simulink model "ball_and_plate_za_nn_2"  (R2018b)
settings: Solver=ode45  StartTime=0.0  StopTime=t_sim  RelTol=1e-3  EnableMultiTasking=on
values from neighbouring files (symbols this model uses):
  A_x = 0.05    [parametri.mat]    (also in proba_nn_simulink.m = 0.1; simulate_NOE_NARX_performance.mat = 0.1; simuliraj_kruznicu.m = radijus; test_nn_.m = 0.1)
  a_x = 0.388    [parametri.mat]    (also in simulate_NOE_NARX_performance.mat)
  A_y = 0.05    [parametri.mat]    (also in proba_nn_simulink.m = 0.1; simulate_NOE_NARX_performance.mat = 0.1; simuliraj_kruznicu.m = radijus; test_nn_.m = 0.1)
  a_y = 0.473    [parametri.mat]    (also in simulate_NOE_NARX_performance.mat)
  Ak_x = 0.1    [parametri.mat]    (also in simulate_NOE_NARX_performance.mat; simuliraj_kvadrat.m = stranica)
  Ak_y = 0.1    [parametri.mat]    (also in simulate_NOE_NARX_performance.mat; simuliraj_kvadrat.m = stranica)
  d = 2    [parametri.mat]    (also in simulate_NOE_NARX_performance.mat)
  Fc = 9.9675e-08    [parametri.mat]    (also in simulate_NOE_NARX_performance.mat)
  freq_x = 0.628318530718    [parametri.mat]    (also in simulate_NOE_NARX_performance.mat)
  freq_y = 0.628318530718    [parametri.mat]    (also in simulate_NOE_NARX_performance.mat)
  Fs = 1.9935e-07    [parametri.mat]    (also in simulate_NOE_NARX_performance.mat)
  g = 9.81    [parametri.mat]    (also in simulate_NOE_NARX_performance.mat)
  Jl = 7.48815837481e-05    [parametri.mat]    (also in simulate_NOE_NARX_performance.mat)
  konstanta = 0.1    [parametri.mat]    (also in simulate_NOE_NARX_performance.mat; simuliraj_kvadrat.m = 0.03)
  l = 0.1    [parametri.mat]    (also in simulate_NOE_NARX_performance.mat)
  ml = 0.0786597330257    [parametri.mat]    (also in simulate_NOE_NARX_performance.mat)
  odabir = 3    [proba_nn_simulink.m]    (also in simulate_NOE_NARX_performance.mat; simuliraj_kruznicu.m; simuliraj_kvadrat.m = 2; simuliraj_referenca.m = 1)
  period_x = 16    [parametri.mat]    (also in simulate_NOE_NARX_performance.mat)
  period_y = 16    [parametri.mat]    (also in simulate_NOE_NARX_performance.mat)
  phase_x = 1.57079632679    [parametri.mat]    (also in simulate_NOE_NARX_performance.mat)
  phase_y = 0    [parametri.mat]    (also in simulate_NOE_NARX_performance.mat)
  phasedelay_x = 0    [parametri.mat]    (also in simulate_NOE_NARX_performance.mat)
  phasedelay_y = 4    [parametri.mat]    (also in simulate_NOE_NARX_performance.mat)
  pw_x = 50    [parametri.mat]    (also in simulate_NOE_NARX_performance.mat)
  pw_y = 50    [parametri.mat]    (also in simulate_NOE_NARX_performance.mat)
  R = 0.0397    [parametri.mat]    (also in simulate_NOE_NARX_performance.mat)
  r = 0.02    [parametri.mat]    (also in simulate_NOE_NARX_performance.mat)
  t_step = 5    [parametri.mat]    (also in simulate_NOE_NARX_performance.mat)
  Td = 0.1    [parametri.mat]    (also in simulate_NOE_NARX_performance.mat)
  vs = 0.05    [parametri.mat]    (also in simulate_NOE_NARX_performance.mat)
  x0 = 0.15    [parametri.mat]    (also in proba_nn_simulink.m = a_x/2.0; simulate_NOE_NARX_performance.mat = 0.194; simuliraj_kruznicu.m = a_x/2.0; test_nn_.m = a_x/2.0)
  x0_loptica = 0.1    [proba_nn_simulink.m]    (also in simulate_NOE_NARX_performance.mat; simuliraj_kruznicu.m = x0_poc; simuliraj_kvadrat.m = x0_poc; simuliraj_referenca.m = x0_poc)
  x_step = 0.05    [parametri.mat]    (also in simulate_NOE_NARX_performance.mat; simuliraj_referenca.m = x_ref_value)
  y0 = 0.15    [parametri.mat]    (also in proba_nn_simulink.m = a_y/2.0; simulate_NOE_NARX_performance.mat = 0.2365; simuliraj_kruznicu.m = a_y/2.0; test_nn_.m = a_y/2.0)
  y0_loptica = 0.1    [proba_nn_simulink.m]    (also in simulate_NOE_NARX_performance.mat; simuliraj_kruznicu.m = y0_poc; simuliraj_kvadrat.m = y0_poc; simuliraj_referenca.m = y0_poc)
  y_step = 0.05    [parametri.mat]    (also in simulate_NOE_NARX_performance.mat; simuliraj_referenca.m = y_ref_value)
libraries: neural x118, simulink x6, fuzblock x2
(part 4 of 5)

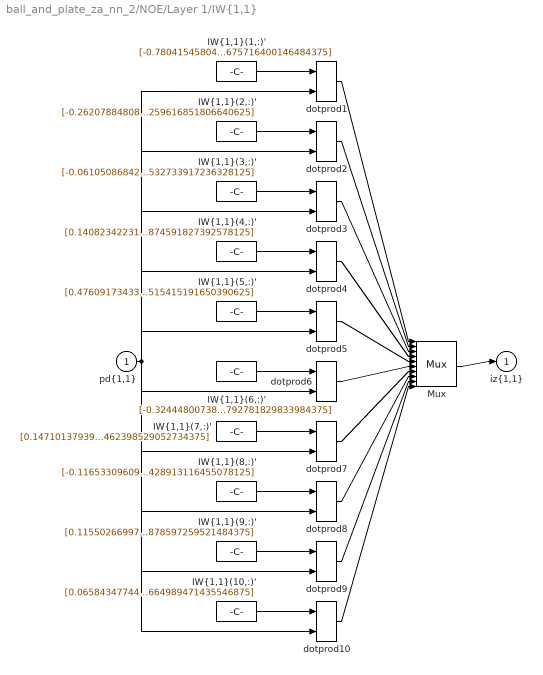
== system ball_and_plate_za_nn_2/NOE/Layer 1/IW{1,1} ==
  "pd{1,1}" : Inport  PortDimensions=5  SampleTime=0.001
      mask Display: e = 0.06;c1 = [120 230 180]/255;c2 = ([120 230 180]+0)/(256+128);c3 = ([120 230 180]+128)/(256+128);patch([0 1 1 0],[0 0 1 1],c1);patch([0 1 1 1-e 1-e 0+e],[0 0 1 1-e 0+e 0+e],c2);patch([0 0 1 1-e 0+e 0+e],[0 1 1 1-e 1-e 0+e],c3);plot([0 1 1 0 0],[0 0 1 1 0]);
  "IW{1,1}(1,:)'" : Constant  Value=[-0.78041545804284273568640628582215867936611175537109375;-0.1889168057158937263917408699853694997727870941162109375;0.624203755586431707769179411116056144237518310546875;0.38254385586967643018141416177968494594097137451171875;0.11132858481816297613331556703997193835675716400146484375]
      mask Display: e = 0.06;c1 = [120 150 230]/255;c2 = ([120 150 230]+0)/383;c3 = ([120 150 230]+128)/383;patch([0 1 1 0],[0 0 1 1],c1);patch([0 1 1 1-e 1-e 0+e],[0 0 1 1-e 0+e 0+e],c2);patch([0 0 1 1-e 0+e 0+e],[0 1 1 1-e 1-e 0+e],c3);plot([0 1 1 0 0],[0 0 1 1 0]);disp('Weights');
  "IW{1,1}(10,:)'" : Constant  Value=[0.06584347744638797961247433931930572725832462310791015625;-0.14742080631494014486548849163227714598178863525390625;-0.449429553740740950207310788755421526730060577392578125;-0.10537733622991619919506689484478556551039218902587890625;0.57322556196782226134445181742194108664989471435546875]
      mask Display: e = 0.06;c1 = [120 150 230]/255;c2 = ([120 150 230]+0)/383;c3 = ([120 150 230]+128)/383;patch([0 1 1 0],[0 0 1 1],c1);patch([0 1 1 1-e 1-e 0+e],[0 0 1 1-e 0+e 0+e],c2);patch([0 0 1 1-e 0+e 0+e],[0 1 1 1-e 1-e 0+e],c3);plot([0 1 1 0 0],[0 0 1 1 0]);disp('Weights');
  "IW{1,1}(2,:)'" : Constant  Value=[-0.26207884808871162451993086506263352930545806884765625;0.06367181522086796940929076527027064003050327301025390625;0.06797795577746899853277540159979253076016902923583984375;0.469471262437006375822790005258866585791110992431640625;0.196872246361272262848984837546595372259616851806640625]
      mask Display: e = 0.06;c1 = [120 150 230]/255;c2 = ([120 150 230]+0)/383;c3 = ([120 150 230]+128)/383;patch([0 1 1 0],[0 0 1 1],c1);patch([0 1 1 1-e 1-e 0+e],[0 0 1 1-e 0+e 0+e],c2);patch([0 0 1 1-e 0+e 0+e],[0 1 1 1-e 1-e 0+e],c3);plot([0 1 1 0 0],[0 0 1 1 0]);disp('Weights');
  "IW{1,1}(3,:)'" : Constant  Value=[-0.06105086842811814629161659695455455221235752105712890625;0.4362035008337665775712821414344944059848785400390625;0.4757244892843950356819959779386408627033233642578125;-0.332950625751637419025286135365604422986507415771484375;-0.1849610518275301984658653964288532733917236328125]
      mask Display: e = 0.06;c1 = [120 150 230]/255;c2 = ([120 150 230]+0)/383;c3 = ([120 150 230]+128)/383;patch([0 1 1 0],[0 0 1 1],c1);patch([0 1 1 1-e 1-e 0+e],[0 0 1 1-e 0+e 0+e],c2);patch([0 0 1 1-e 0+e 0+e],[0 1 1 1-e 1-e 0+e],c3);plot([0 1 1 0 0],[0 0 1 1 0]);disp('Weights');
  "IW{1,1}(4,:)'" : Constant  Value=[0.1408234223110425842317994238328537903726100921630859375;-0.13205465366012736350143086383468471467494964599609375;-0.493931339703755745151880773846642114222049713134765625;-0.2126283255869568511453593373516923747956752777099609375;-0.12407140487677166540425588436846737749874591827392578125]
      mask Display: e = 0.06;c1 = [120 150 230]/255;c2 = ([120 150 230]+0)/383;c3 = ([120 150 230]+128)/383;patch([0 1 1 0],[0 0 1 1],c1);patch([0 1 1 1-e 1-e 0+e],[0 0 1 1-e 0+e 0+e],c2);patch([0 0 1 1-e 0+e 0+e],[0 1 1 1-e 1-e 0+e],c3);plot([0 1 1 0 0],[0 0 1 1 0]);disp('Weights');
  "IW{1,1}(5,:)'" : Constant  Value=[0.476091734332447114041997338063083589076995849609375;-0.63150999375165917104624213607166893780231475830078125;-0.515564815245219687511735173757188022136688232421875;-0.1465624758355017487332361270091496407985687255859375;0.2165017929034026844536953149145119823515415191650390625]
      mask Display: e = 0.06;c1 = [120 150 230]/255;c2 = ([120 150 230]+0)/383;c3 = ([120 150 230]+128)/383;patch([0 1 1 0],[0 0 1 1],c1);patch([0 1 1 1-e 1-e 0+e],[0 0 1 1-e 0+e 0+e],c2);patch([0 0 1 1-e 0+e 0+e],[0 1 1 1-e 1-e 0+e],c3);plot([0 1 1 0 0],[0 0 1 1 0]);disp('Weights');
  "IW{1,1}(6,:)'" : Constant  Value=[-0.324448007382350411820226554482360370457172393798828125;-0.166002451601267642100623334044939838349819183349609375;0.297221055954937696252926571105490438640117645263671875;0.380975071646488083754178433082415722310543060302734375;-0.233386025845927436161986179286031983792781829833984375]
      mask Display: e = 0.06;c1 = [120 150 230]/255;c2 = ([120 150 230]+0)/383;c3 = ([120 150 230]+128)/383;patch([0 1 1 0],[0 0 1 1],c1);patch([0 1 1 1-e 1-e 0+e],[0 0 1 1-e 0+e 0+e],c2);patch([0 0 1 1-e 0+e 0+e],[0 1 1 1-e 1-e 0+e],c3);plot([0 1 1 0 0],[0 0 1 1 0]);disp('Weights');
  "IW{1,1}(7,:)'" : Constant  Value=[0.1471013793978408756846221194791723974049091339111328125;-0.039050046429146945126120726854423992335796356201171875;0.441337535111876066995506562307127751410007476806640625;0.1489052345501019336548864657743251882493495941162109375;0.01257927307039984066161508735604002140462398529052734375]
      mask Display: e = 0.06;c1 = [120 150 230]/255;c2 = ([120 150 230]+0)/383;c3 = ([120 150 230]+128)/383;patch([0 1 1 0],[0 0 1 1],c1);patch([0 1 1 1-e 1-e 0+e],[0 0 1 1-e 0+e 0+e],c2);patch([0 0 1 1-e 0+e 0+e],[0 1 1 1-e 1-e 0+e],c3);plot([0 1 1 0 0],[0 0 1 1 0]);disp('Weights');
  "IW{1,1}(8,:)'" : Constant  Value=[-0.11653309609751634490226734897078131325542926788330078125;0.377889179667925290129204540789942257106304168701171875;0.2200242920649362332596865599043667316436767578125;-0.07683035892270144440185930534426006488502025604248046875;0.462132111220164620846162506495602428913116455078125]
      mask Display: e = 0.06;c1 = [120 150 230]/255;c2 = ([120 150 230]+0)/383;c3 = ([120 150 230]+128)/383;patch([0 1 1 0],[0 0 1 1],c1);patch([0 1 1 1-e 1-e 0+e],[0 0 1 1-e 0+e 0+e],c2);patch([0 0 1 1-e 0+e 0+e],[0 1 1 1-e 1-e 0+e],c3);plot([0 1 1 0 0],[0 0 1 1 0]);disp('Weights');
  "IW{1,1}(9,:)'" : Constant  Value=[0.11550266997215274944466045781155116856098175048828125;0.387383375581388078590094892206252552568912506103515625;-0.62457516979531668699365809516166336834430694580078125;-0.0744787101351869207377376369549892842769622802734375;0.83112863904779332724359619533061049878597259521484375]
      mask Display: e = 0.06;c1 = [120 150 230]/255;c2 = ([120 150 230]+0)/383;c3 = ([120 150 230]+128)/383;patch([0 1 1 0],[0 0 1 1],c1);patch([0 1 1 1-e 1-e 0+e],[0 0 1 1-e 0+e 0+e],c2);patch([0 0 1 1-e 0+e 0+e],[0 1 1 1-e 1-e 0+e],c3);plot([0 1 1 0 0],[0 0 1 1 0]);disp('Weights');
  Mux : Mux  Inputs=10
      mask Display: e = 0.06;c1 = [120 150 230]/255;c2 = ([120 150 230]+0)/383;c3 = ([120 150 230]+128)/383;patch([0 1 1 0],[0 0 1 1],c1);patch([0 1 1 1-e 1-e 0+e],[0 0 1 1-e 0+e 0+e],c2);patch([0 0 1 1-e 0+e 0+e],[0 1 1 1-e 1-e 0+e],c3);plot([0 1 1 0 0],[0 0 1 1 0]);disp('Mux');
  dotprod{1..10} (10 alike) : neural/Weight Functions/dotprod
  "iz{1,1}" : Outport
      mask Display: e = 0.06;c1 = [120 230 180]/255;c2 = ([120 230 180]+0)/(256+128);c3 = ([120 230 180]+128)/(256+128);patch([0 1 1 0],[0 0 1 1],c1);patch([0 1 1 1-e 1-e 0+e],[0 0 1 1-e 0+e 0+e],c2);patch([0 0 1 1-e 0+e 0+e],[0 1 1 1-e 1-e 0+e],c3);plot([0 1 1 0 0],[0 0 1 1 0]);
  wires:
  "IW{1,1}(1,:)'"/1 -> dotprod1/1
  "pd{1,1}"/1 -> dotprod1/2, dotprod2/2, dotprod3/2, dotprod4/2, dotprod5/2, dotprod6/2, dotprod7/2, dotprod8/2, dotprod9/2, dotprod10/2
  dotprod1/1 -> Mux/1
  "IW{1,1}(2,:)'"/1 -> dotprod2/1
  dotprod2/1 -> Mux/2
  "IW{1,1}(3,:)'"/1 -> dotprod3/1
  dotprod3/1 -> Mux/3
  "IW{1,1}(4,:)'"/1 -> dotprod4/1
  dotprod4/1 -> Mux/4
  "IW{1,1}(5,:)'"/1 -> dotprod5/1
  dotprod5/1 -> Mux/5
  "IW{1,1}(6,:)'"/1 -> dotprod6/1
  dotprod6/1 -> Mux/6
  "IW{1,1}(7,:)'"/1 -> dotprod7/1
  dotprod7/1 -> Mux/7
  "IW{1,1}(8,:)'"/1 -> dotprod8/1
  dotprod8/1 -> Mux/8
  "IW{1,1}(9,:)'"/1 -> dotprod9/1
  dotprod9/1 -> Mux/9
  "IW{1,1}(10,:)'"/1 -> dotprod10/1
  dotprod10/1 -> Mux/10
  Mux/1 -> "iz{1,1}"/1

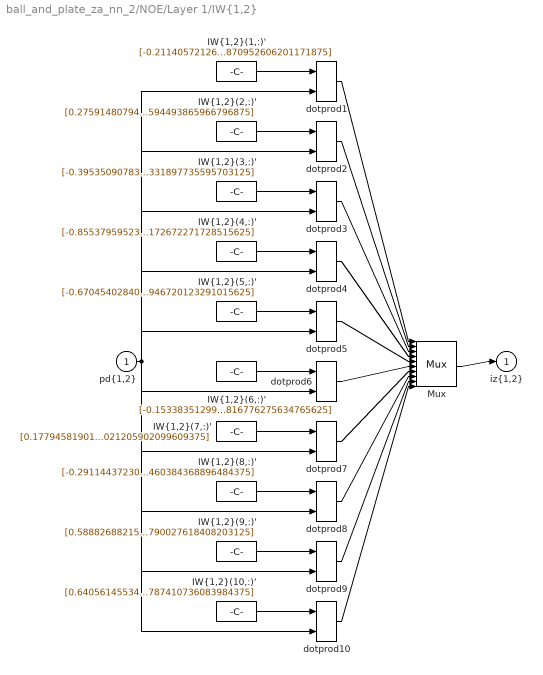
== system ball_and_plate_za_nn_2/NOE/Layer 1/IW{1,2} ==
  "pd{1,2}" : Inport  PortDimensions=5  SampleTime=0.001
      mask Display: e = 0.06;c1 = [120 230 180]/255;c2 = ([120 230 180]+0)/(256+128);c3 = ([120 230 180]+128)/(256+128);patch([0 1 1 0],[0 0 1 1],c1);patch([0 1 1 1-e 1-e 0+e],[0 0 1 1-e 0+e 0+e],c2);patch([0 0 1 1-e 0+e 0+e],[0 1 1 1-e 1-e 0+e],c3);plot([0 1 1 0 0],[0 0 1 1 0]);
  "IW{1,2}(1,:)'" : Constant  Value=[-0.211405721260622792012640047687455080449581146240234375;0.9834201495236669643418281339108943939208984375;0.078318433789418495649670148850418627262115478515625;0.62573603116239862043101993549498729407787322998046875;-0.4606972890689788879825528056244365870952606201171875]
      mask Display: e = 0.06;c1 = [120 150 230]/255;c2 = ([120 150 230]+0)/383;c3 = ([120 150 230]+128)/383;patch([0 1 1 0],[0 0 1 1],c1);patch([0 1 1 1-e 1-e 0+e],[0 0 1 1-e 0+e 0+e],c2);patch([0 0 1 1-e 0+e 0+e],[0 1 1 1-e 1-e 0+e],c3);plot([0 1 1 0 0],[0 0 1 1 0]);disp('Weights');
  "IW{1,2}(10,:)'" : Constant  Value=[0.64056145534157327148250260506756603717803955078125;0.600565723799352024769859781372360885143280029296875;0.2156582058706855153928927393280901014804840087890625;0.6943897986555647161566184877301566302776336669921875;-0.60339661147887768688491405555396340787410736083984375]
      mask Display: e = 0.06;c1 = [120 150 230]/255;c2 = ([120 150 230]+0)/383;c3 = ([120 150 230]+128)/383;patch([0 1 1 0],[0 0 1 1],c1);patch([0 1 1 1-e 1-e 0+e],[0 0 1 1-e 0+e 0+e],c2);patch([0 0 1 1-e 0+e 0+e],[0 1 1 1-e 1-e 0+e],c3);plot([0 1 1 0 0],[0 0 1 1 0]);disp('Weights');
  "IW{1,2}(2,:)'" : Constant  Value=[0.2759148079449758039771722906152717769145965576171875;-0.42325449718057639447721385295153595507144927978515625;-0.1532778579257629003596008487875224091112613677978515625;-0.482010946294399167388888827190385200083255767822265625;-0.664216850422650662011392341810278594493865966796875]
      mask Display: e = 0.06;c1 = [120 150 230]/255;c2 = ([120 150 230]+0)/383;c3 = ([120 150 230]+128)/383;patch([0 1 1 0],[0 0 1 1],c1);patch([0 1 1 1-e 1-e 0+e],[0 0 1 1-e 0+e 0+e],c2);patch([0 0 1 1-e 0+e 0+e],[0 1 1 1-e 1-e 0+e],c3);plot([0 1 1 0 0],[0 0 1 1 0]);disp('Weights');
  "IW{1,2}(3,:)'" : Constant  Value=[-0.39535090783148596482732273216242901980876922607421875;0.0030548046006235456302502218051131421816535294055938720703125;-0.381754713214691510092535509102162905037403106689453125;-0.137371181736283987095958991631050594151020050048828125;-0.54520998452879265716575218903017230331897735595703125]
      mask Display: e = 0.06;c1 = [120 150 230]/255;c2 = ([120 150 230]+0)/383;c3 = ([120 150 230]+128)/383;patch([0 1 1 0],[0 0 1 1],c1);patch([0 1 1 1-e 1-e 0+e],[0 0 1 1-e 0+e 0+e],c2);patch([0 0 1 1-e 0+e 0+e],[0 1 1 1-e 1-e 0+e],c3);plot([0 1 1 0 0],[0 0 1 1 0]);disp('Weights');
  "IW{1,2}(4,:)'" : Constant  Value=[-0.85537959523864859345820832459139637649059295654296875;-0.003498486669252578139255316358458003378473222255706787109375;0.229525682886273785232589261795510537922382354736328125;-0.69954557852212229107635721447877585887908935546875;0.003780760113263581002895907801075736642815172672271728515625]
      mask Display: e = 0.06;c1 = [120 150 230]/255;c2 = ([120 150 230]+0)/383;c3 = ([120 150 230]+128)/383;patch([0 1 1 0],[0 0 1 1],c1);patch([0 1 1 1-e 1-e 0+e],[0 0 1 1-e 0+e 0+e],c2);patch([0 0 1 1-e 0+e 0+e],[0 1 1 1-e 1-e 0+e],c3);plot([0 1 1 0 0],[0 0 1 1 0]);disp('Weights');
  "IW{1,2}(5,:)'" : Constant  Value=[-0.6704540284077300515974684458342380821704864501953125;-0.1356854228754304225734728106544935144484043121337890625;-0.668394792329869869007552551920525729656219482421875;0.44352275149486819483257704632706008851528167724609375;0.1269145397078425274717261572732240892946720123291015625]
      mask Display: e = 0.06;c1 = [120 150 230]/255;c2 = ([120 150 230]+0)/383;c3 = ([120 150 230]+128)/383;patch([0 1 1 0],[0 0 1 1],c1);patch([0 1 1 1-e 1-e 0+e],[0 0 1 1-e 0+e 0+e],c2);patch([0 0 1 1-e 0+e 0+e],[0 1 1 1-e 1-e 0+e],c3);plot([0 1 1 0 0],[0 0 1 1 0]);disp('Weights');
  "IW{1,2}(6,:)'" : Constant  Value=[-0.153383512992241455297204311136738397181034088134765625;-0.1582862661763130562864176908988156355917453765869140625;-0.2420745637484461865174267813927144743502140045166015625;-0.574128226120135476406858288100920617580413818359375;-0.60140197031635145297201461289660073816776275634765625]
      mask Display: e = 0.06;c1 = [120 150 230]/255;c2 = ([120 150 230]+0)/383;c3 = ([120 150 230]+128)/383;patch([0 1 1 0],[0 0 1 1],c1);patch([0 1 1 1-e 1-e 0+e],[0 0 1 1-e 0+e 0+e],c2);patch([0 0 1 1-e 0+e 0+e],[0 1 1 1-e 1-e 0+e],c3);plot([0 1 1 0 0],[0 0 1 1 0]);disp('Weights');
  "IW{1,2}(7,:)'" : Constant  Value=[0.1779458190130129568995442923551308922469615936279296875;0.79003871229958788635627797702909447252750396728515625;0.4392010876973493349595401014084927737712860107421875;0.51372629645238532258844088573823682963848114013671875;0.2078732017274463605982504077474004589021205902099609375]
      mask Display: e = 0.06;c1 = [120 150 230]/255;c2 = ([120 150 230]+0)/383;c3 = ([120 150 230]+128)/383;patch([0 1 1 0],[0 0 1 1],c1);patch([0 1 1 1-e 1-e 0+e],[0 0 1 1-e 0+e 0+e],c2);patch([0 0 1 1-e 0+e 0+e],[0 1 1 1-e 1-e 0+e],c3);plot([0 1 1 0 0],[0 0 1 1 0]);disp('Weights');
  "IW{1,2}(8,:)'" : Constant  Value=[-0.29114437230780498833127012403565458953380584716796875;-0.7687057090658928615312106558121740818023681640625;0.1507041762917487315309728046486270613968372344970703125;-0.3169104871757533192777600561385042965412139892578125;0.475119755527989739984917605397640727460384368896484375]
      mask Display: e = 0.06;c1 = [120 150 230]/255;c2 = ([120 150 230]+0)/383;c3 = ([120 150 230]+128)/383;patch([0 1 1 0],[0 0 1 1],c1);patch([0 1 1 1-e 1-e 0+e],[0 0 1 1-e 0+e 0+e],c2);patch([0 0 1 1-e 0+e 0+e],[0 1 1 1-e 1-e 0+e],c3);plot([0 1 1 0 0],[0 0 1 1 0]);disp('Weights');
  "IW{1,2}(9,:)'" : Constant  Value=[0.58882688215316736357607396712410263717174530029296875;-0.10413231615864219914424637636329862289130687713623046875;0.16252337571316655129294304060749709606170654296875;0.2493172541404560238476051381439901888370513916015625;-1.0104188868762673525480977332335896790027618408203125]
      mask Display: e = 0.06;c1 = [120 150 230]/255;c2 = ([120 150 230]+0)/383;c3 = ([120 150 230]+128)/383;patch([0 1 1 0],[0 0 1 1],c1);patch([0 1 1 1-e 1-e 0+e],[0 0 1 1-e 0+e 0+e],c2);patch([0 0 1 1-e 0+e 0+e],[0 1 1 1-e 1-e 0+e],c3);plot([0 1 1 0 0],[0 0 1 1 0]);disp('Weights');
  Mux : Mux  Inputs=10
      mask Display: e = 0.06;c1 = [120 150 230]/255;c2 = ([120 150 230]+0)/383;c3 = ([120 150 230]+128)/383;patch([0 1 1 0],[0 0 1 1],c1);patch([0 1 1 1-e 1-e 0+e],[0 0 1 1-e 0+e 0+e],c2);patch([0 0 1 1-e 0+e 0+e],[0 1 1 1-e 1-e 0+e],c3);plot([0 1 1 0 0],[0 0 1 1 0]);disp('Mux');
  dotprod{1..10} (10 alike) : neural/Weight Functions/dotprod
  "iz{1,2}" : Outport
      mask Display: e = 0.06;c1 = [120 230 180]/255;c2 = ([120 230 180]+0)/(256+128);c3 = ([120 230 180]+128)/(256+128);patch([0 1 1 0],[0 0 1 1],c1);patch([0 1 1 1-e 1-e 0+e],[0 0 1 1-e 0+e 0+e],c2);patch([0 0 1 1-e 0+e 0+e],[0 1 1 1-e 1-e 0+e],c3);plot([0 1 1 0 0],[0 0 1 1 0]);
  wires:
  "IW{1,2}(1,:)'"/1 -> dotprod1/1
  "pd{1,2}"/1 -> dotprod1/2, dotprod2/2, dotprod3/2, dotprod4/2, dotprod5/2, dotprod6/2, dotprod7/2, dotprod8/2, dotprod9/2, dotprod10/2
  dotprod1/1 -> Mux/1
  "IW{1,2}(2,:)'"/1 -> dotprod2/1
  dotprod2/1 -> Mux/2
  "IW{1,2}(3,:)'"/1 -> dotprod3/1
  dotprod3/1 -> Mux/3
  "IW{1,2}(4,:)'"/1 -> dotprod4/1
  dotprod4/1 -> Mux/4
  "IW{1,2}(5,:)'"/1 -> dotprod5/1
  dotprod5/1 -> Mux/5
  "IW{1,2}(6,:)'"/1 -> dotprod6/1
  dotprod6/1 -> Mux/6
  "IW{1,2}(7,:)'"/1 -> dotprod7/1
  dotprod7/1 -> Mux/7
  "IW{1,2}(8,:)'"/1 -> dotprod8/1
  dotprod8/1 -> Mux/8
  "IW{1,2}(9,:)'"/1 -> dotprod9/1
  dotprod9/1 -> Mux/9
  "IW{1,2}(10,:)'"/1 -> dotprod10/1
  dotprod10/1 -> Mux/10
  Mux/1 -> "iz{1,2}"/1

== system ball_and_plate_za_nn_2/NOE/Layer 2/Delays 1 ==
  "p{2}" : Inport  PortDimensions=10  SampleTime=0.001
      mask Display: e = 0.06;c1 = [120 230 180]/255;c2 = ([120 230 180]+0)/(256+128);c3 = ([120 230 180]+128)/(256+128);patch([0 1 1 0],[0 0 1 1],c1);patch([0 1 1 1-e 1-e 0+e],[0 0 1 1-e 0+e 0+e],c2);patch([0 0 1 1-e 0+e 0+e],[0 1 1 1-e 1-e 0+e],c3);plot([0 1 1 0 0],[0 0 1 1 0]);
  mux : Mux  Inputs=1
      mask Display: e = 0.06;c1 = [120 150 230]/255;c2 = ([120 150 230]+0)/383;c3 = ([120 150 230]+128)/383;patch([0 1 1 0],[0 0 1 1],c1);patch([0 1 1 1-e 1-e 0+e],[0 0 1 1-e 0+e 0+e],c2);patch([0 0 1 1-e 0+e 0+e],[0 1 1 1-e 1-e 0+e],c3);plot([0 1 1 0 0],[0 0 1 1 0]);disp('Mux')
  "pd{2,1}" : Outport
      mask Display: e = 0.06;c1 = [120 230 180]/255;c2 = ([120 230 180]+0)/(256+128);c3 = ([120 230 180]+128)/(256+128);patch([0 1 1 0],[0 0 1 1],c1);patch([0 1 1 1-e 1-e 0+e],[0 0 1 1-e 0+e 0+e],c2);patch([0 0 1 1-e 0+e 0+e],[0 1 1 1-e 1-e 0+e],c3);plot([0 1 1 0 0],[0 0 1 1 0]);
  wires:
  "p{2}"/1 -> mux/1
  mux/1 -> "pd{2,1}"/1

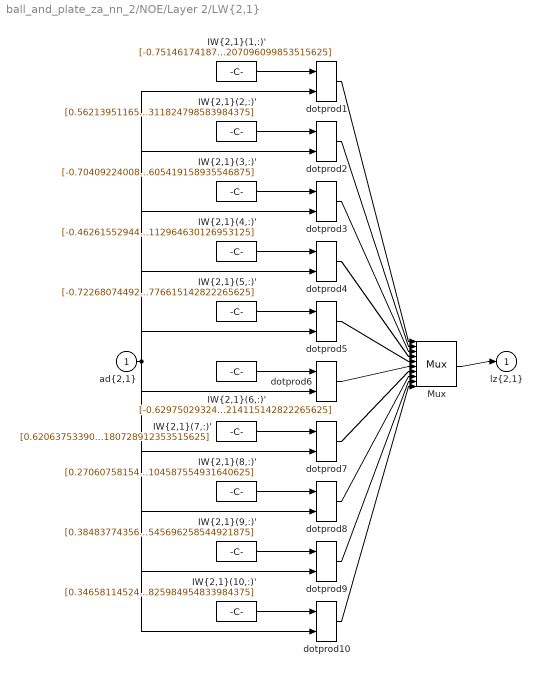
== system ball_and_plate_za_nn_2/NOE/Layer 2/LW{2,1} ==
  "ad{2,1}" : Inport  PortDimensions=10  SampleTime=0.001
      mask Display: e = 0.06;c1 = [120 230 180]/255;c2 = ([120 230 180]+0)/(256+128);c3 = ([120 230 180]+128)/(256+128);patch([0 1 1 0],[0 0 1 1],c1);patch([0 1 1 1-e 1-e 0+e],[0 0 1 1-e 0+e 0+e],c2);patch([0 0 1 1-e 0+e 0+e],[0 1 1 1-e 1-e 0+e],c3);plot([0 1 1 0 0],[0 0 1 1 0]);
  "IW{2,1}(1,:)'" : Constant  Value=[-0.751461741877256894639458550955168902873992919921875;0.01402301635471886638584226858483816613443195819854736328125;0.326442792203841147813392353782546706497669219970703125;0.90660022935466921811809015707694925367832183837890625;-0.407952329174343153450621457523084245622158050537109375;0.609601578751406858458494752994738519191741943359375;-0.255621626399888779435087826641392894089221954345703125;0.10066722871003118411348253857795498333871364593505859375;0.64998266078069499851466161999269388616085052490234375;0.0938512522285636363594818476485670544207096099853515625]
      mask Display: e = 0.06;c1 = [120 150 230]/255;c2 = ([120 150 230]+0)/383;c3 = ([120 150 230]+128)/383;patch([0 1 1 0],[0 0 1 1],c1);patch([0 1 1 1-e 1-e 0+e],[0 0 1 1-e 0+e 0+e],c2);patch([0 0 1 1-e 0+e 0+e],[0 1 1 1-e 1-e 0+e],c3);plot([0 1 1 0 0],[0 0 1 1 0]);disp('weights');
  "IW{2,1}(10,:)'" : Constant  Value=[0.346581145248940847292118405675864778459072113037109375;-0.101987596917314904398921271422295831143856048583984375;-0.199988337664544435501312591441092081367969512939453125;-0.0897556143633064795750442499411292374134063720703125;-0.194407172548844597859130090000689961016178131103515625;-0.8538132542041305672597673037671484053134918212890625;-0.57795138239333410101750132525921799242496490478515625;-0.75194724899415821273152005232986994087696075439453125;-0.5683703056683737653287380453548394143581390380859375;-0.86428952174772832872662320369272492825984954833984375]
      mask Display: e = 0.06;c1 = [120 150 230]/255;c2 = ([120 150 230]+0)/383;c3 = ([120 150 230]+128)/383;patch([0 1 1 0],[0 0 1 1],c1);patch([0 1 1 1-e 1-e 0+e],[0 0 1 1-e 0+e 0+e],c2);patch([0 0 1 1-e 0+e 0+e],[0 1 1 1-e 1-e 0+e],c3);plot([0 1 1 0 0],[0 0 1 1 0]);disp('weights');
  "IW{2,1}(2,:)'" : Constant  Value=[0.56213951165120590314216997285257093608379364013671875;-0.40896438246015787143505804124288260936737060546875;-0.273757397181592476709255379319074563682079315185546875;-0.3103497860711339484396376064978539943695068359375;0.280879223850993786637531002270407043397426605224609375;0.89661471211202348197133460416807793080806732177734375;-0.340117465515137384901578343487926758825778961181640625;-0.249746831523702639277217940616537816822528839111328125;0.572224831191468386037968230084516108036041259765625;0.8546385328160768235505884149461053311824798583984375]
      mask Display: e = 0.06;c1 = [120 150 230]/255;c2 = ([120 150 230]+0)/383;c3 = ([120 150 230]+128)/383;patch([0 1 1 0],[0 0 1 1],c1);patch([0 1 1 1-e 1-e 0+e],[0 0 1 1-e 0+e 0+e],c2);patch([0 0 1 1-e 0+e 0+e],[0 1 1 1-e 1-e 0+e],c3);plot([0 1 1 0 0],[0 0 1 1 0]);disp('weights');
  "IW{2,1}(3,:)'" : Constant  Value=[-0.70409224008847426379276157604181207716464996337890625;0.437857221912158312004947902096319012343883514404296875;0.387908650182214154167326114475145004689693450927734375;-0.313310564539420910445954859824269078671932220458984375;0.5966351041570219226883864394039846956729888916015625;0.25544146338399542628394556231796741485595703125;0.1801270507966407918853946057424764148890972137451171875;-0.1924515838328022809822215322128613479435443878173828125;1.0313756586178184360136356190196238458156585693359375;-0.2004747683477036968024975749358418397605419158935546875]
      mask Display: e = 0.06;c1 = [120 150 230]/255;c2 = ([120 150 230]+0)/383;c3 = ([120 150 230]+128)/383;patch([0 1 1 0],[0 0 1 1],c1);patch([0 1 1 1-e 1-e 0+e],[0 0 1 1-e 0+e 0+e],c2);patch([0 0 1 1-e 0+e 0+e],[0 1 1 1-e 1-e 0+e],c3);plot([0 1 1 0 0],[0 0 1 1 0]);disp('weights');
  "IW{2,1}(4,:)'" : Constant  Value=[-0.46261552944577744028720189817249774932861328125;-0.6083303245955329341398964970721863210201263427734375;0.381563465677544011445121441283845342695713043212890625;0.80056607469864016213279001021874137222766876220703125;0.114817651105901308294932050557690672576427459716796875;-0.31942984216014080889323167866677977144718170166015625;-0.3081261823478540495813149391324259340763092041015625;-0.806724202034220905233041776227764785289764404296875;-0.707544236757142730454006596119143068790435791015625;0.353957390817320860509909152824548073112964630126953125]
      mask Display: e = 0.06;c1 = [120 150 230]/255;c2 = ([120 150 230]+0)/383;c3 = ([120 150 230]+128)/383;patch([0 1 1 0],[0 0 1 1],c1);patch([0 1 1 1-e 1-e 0+e],[0 0 1 1-e 0+e 0+e],c2);patch([0 0 1 1-e 0+e 0+e],[0 1 1 1-e 1-e 0+e],c3);plot([0 1 1 0 0],[0 0 1 1 0]);disp('weights');
  "IW{2,1}(5,:)'" : Constant  Value=[-0.72268074492281775267343846280709840357303619384765625;-0.8099425973058613781319081681431271135807037353515625;-0.48012472297759967165831085367244668304920196533203125;-0.374216308436248923374733976743300445377826690673828125;0.32503796485929414838977891122340224683284759521484375;0.6499760510715775208012701114057563245296478271484375;0.1020332046731853570253889529340085573494434356689453125;-0.51431091597126921133309451761306263506412506103515625;0.2133497896093230483671732145012356340885162353515625;-0.191885414877650595233404828832135535776615142822265625]
      mask Display: e = 0.06;c1 = [120 150 230]/255;c2 = ([120 150 230]+0)/383;c3 = ([120 150 230]+128)/383;patch([0 1 1 0],[0 0 1 1],c1);patch([0 1 1 1-e 1-e 0+e],[0 0 1 1-e 0+e 0+e],c2);patch([0 0 1 1-e 0+e 0+e],[0 1 1 1-e 1-e 0+e],c3);plot([0 1 1 0 0],[0 0 1 1 0]);disp('weights');
  "IW{2,1}(6,:)'" : Constant  Value=[-0.629750293245689096721662281197495758533477783203125;-0.66644903841917801923244724093819968402385711669921875;-0.279327203788677869145118393134907819330692291259765625;-0.440689146090105177133722236249013803899288177490234375;0.309771552515399839489163014150108210742473602294921875;0.460903085493117148363495516605325974524021148681640625;-0.22998472818172943643588723716675303876399993896484375;0.07709746790716941189369748599347076378762722015380859375;-0.1743857796929972614474735337353195063769817352294921875;-0.79638649306433484387213184163556434214115142822265625]
      mask Display: e = 0.06;c1 = [120 150 230]/255;c2 = ([120 150 230]+0)/383;c3 = ([120 150 230]+128)/383;patch([0 1 1 0],[0 0 1 1],c1);patch([0 1 1 1-e 1-e 0+e],[0 0 1 1-e 0+e 0+e],c2);patch([0 0 1 1-e 0+e 0+e],[0 1 1 1-e 1-e 0+e],c3);plot([0 1 1 0 0],[0 0 1 1 0]);disp('weights');
  "IW{2,1}(7,:)'" : Constant  Value=[0.620637533906118310511601521284319460391998291015625;0.83539867376766940854082577061490155756473541259765625;0.27920936398507711917460483164177276194095611572265625;0.7752021630701910748229011005605570971965789794921875;-0.52686260303715248820566330323345027863979339599609375;-0.072403514346486785857592849424690939486026763916015625;-0.05991633433839561873046619666638434864580631256103515625;0.5902810493804420133301391615532338619232177734375;-0.57031874551041517040772532709524966776371002197265625;-0.297717100692596103872489265995682217180728912353515625]
      mask Display: e = 0.06;c1 = [120 150 230]/255;c2 = ([120 150 230]+0)/383;c3 = ([120 150 230]+128)/383;patch([0 1 1 0],[0 0 1 1],c1);patch([0 1 1 1-e 1-e 0+e],[0 0 1 1-e 0+e 0+e],c2);patch([0 0 1 1-e 0+e 0+e],[0 1 1 1-e 1-e 0+e],c3);plot([0 1 1 0 0],[0 0 1 1 0]);disp('weights');
  "IW{2,1}(8,:)'" : Constant  Value=[0.27060758154395336827491291842306964099407196044921875;0.608715135034168408623145296587608754634857177734375;0.55085779675167356739251545150182209908962249755859375;-0.51104733314616945794028879390680231153964996337890625;0.07656481679459646583207899084300152026116847991943359375;0.55887912740008005574310345764388330280780792236328125;-0.37549430899164482067220660610473714768886566162109375;-0.7917369512748544391200766767724417150020599365234375;0.08728549133302436480175146016335929743945598602294921875;0.5207839210335978297194969854899682104587554931640625]
      mask Display: e = 0.06;c1 = [120 150 230]/255;c2 = ([120 150 230]+0)/383;c3 = ([120 150 230]+128)/383;patch([0 1 1 0],[0 0 1 1],c1);patch([0 1 1 1-e 1-e 0+e],[0 0 1 1-e 0+e 0+e],c2);patch([0 0 1 1-e 0+e 0+e],[0 1 1 1-e 1-e 0+e],c3);plot([0 1 1 0 0],[0 0 1 1 0]);disp('weights');
  "IW{2,1}(9,:)'" : Constant  Value=[0.384837743561070311226757212352822534739971160888671875;-0.651296741851778104859249651781283318996429443359375;0.2163767641188421020359555768663994967937469482421875;-0.455812576127146484861185626868973486125469207763671875;-0.91015595086147105252649680551257915794849395751953125;-0.79631028649259560925344203496933914721012115478515625;-0.273943343590692334199587776311091147363185882568359375;0.69205197005795648923509588712477125227451324462890625;0.1748269653888369357108700796743505634367465972900390625;-0.2123389122259488892563439321747864596545696258544921875]
      mask Display: e = 0.06;c1 = [120 150 230]/255;c2 = ([120 150 230]+0)/383;c3 = ([120 150 230]+128)/383;patch([0 1 1 0],[0 0 1 1],c1);patch([0 1 1 1-e 1-e 0+e],[0 0 1 1-e 0+e 0+e],c2);patch([0 0 1 1-e 0+e 0+e],[0 1 1 1-e 1-e 0+e],c3);plot([0 1 1 0 0],[0 0 1 1 0]);disp('weights');
  Mux : Mux  Inputs=10
      mask Display: e = 0.06;c1 = [120 150 230]/255;c2 = ([120 150 230]+0)/383;c3 = ([120 150 230]+128)/383;patch([0 1 1 0],[0 0 1 1],c1);patch([0 1 1 1-e 1-e 0+e],[0 0 1 1-e 0+e 0+e],c2);patch([0 0 1 1-e 0+e 0+e],[0 1 1 1-e 1-e 0+e],c3);plot([0 1 1 0 0],[0 0 1 1 0]);disp('Mux');
  dotprod{1..10} (10 alike) : neural/Weight Functions/dotprod
  "lz{2,1}" : Outport
      mask Display: e = 0.06;c1 = [120 230 180]/255;c2 = ([120 230 180]+0)/(256+128);c3 = ([120 230 180]+128)/(256+128);patch([0 1 1 0],[0 0 1 1],c1);patch([0 1 1 1-e 1-e 0+e],[0 0 1 1-e 0+e 0+e],c2);patch([0 0 1 1-e 0+e 0+e],[0 1 1 1-e 1-e 0+e],c3);plot([0 1 1 0 0],[0 0 1 1 0]);
  wires:
  "IW{2,1}(1,:)'"/1 -> dotprod1/1
  "ad{2,1}"/1 -> dotprod1/2, dotprod2/2, dotprod3/2, dotprod4/2, dotprod5/2, dotprod6/2, dotprod7/2, dotprod8/2, dotprod9/2, dotprod10/2
  dotprod1/1 -> Mux/1
  "IW{2,1}(2,:)'"/1 -> dotprod2/1
  dotprod2/1 -> Mux/2
  "IW{2,1}(3,:)'"/1 -> dotprod3/1
  dotprod3/1 -> Mux/3
  "IW{2,1}(4,:)'"/1 -> dotprod4/1
  dotprod4/1 -> Mux/4
  "IW{2,1}(5,:)'"/1 -> dotprod5/1
  dotprod5/1 -> Mux/5
  "IW{2,1}(6,:)'"/1 -> dotprod6/1
  dotprod6/1 -> Mux/6
  "IW{2,1}(7,:)'"/1 -> dotprod7/1
  dotprod7/1 -> Mux/7
  "IW{2,1}(8,:)'"/1 -> dotprod8/1
  dotprod8/1 -> Mux/8
  "IW{2,1}(9,:)'"/1 -> dotprod9/1
  dotprod9/1 -> Mux/9
  "IW{2,1}(10,:)'"/1 -> dotprod10/1
  dotprod10/1 -> Mux/10
  Mux/1 -> "lz{2,1}"/1

== system ball_and_plate_za_nn_2/NOE/Layer 3/Delays 1 ==
  "p{3}" : Inport  PortDimensions=10  SampleTime=0.001
      mask Display: e = 0.06;c1 = [120 230 180]/255;c2 = ([120 230 180]+0)/(256+128);c3 = ([120 230 180]+128)/(256+128);patch([0 1 1 0],[0 0 1 1],c1);patch([0 1 1 1-e 1-e 0+e],[0 0 1 1-e 0+e 0+e],c2);patch([0 0 1 1-e 0+e 0+e],[0 1 1 1-e 1-e 0+e],c3);plot([0 1 1 0 0],[0 0 1 1 0]);
  mux : Mux  Inputs=1
      mask Display: e = 0.06;c1 = [120 150 230]/255;c2 = ([120 150 230]+0)/383;c3 = ([120 150 230]+128)/383;patch([0 1 1 0],[0 0 1 1],c1);patch([0 1 1 1-e 1-e 0+e],[0 0 1 1-e 0+e 0+e],c2);patch([0 0 1 1-e 0+e 0+e],[0 1 1 1-e 1-e 0+e],c3);plot([0 1 1 0 0],[0 0 1 1 0]);disp('Mux')
  "pd{3,2}" : Outport
      mask Display: e = 0.06;c1 = [120 230 180]/255;c2 = ([120 230 180]+0)/(256+128);c3 = ([120 230 180]+128)/(256+128);patch([0 1 1 0],[0 0 1 1],c1);patch([0 1 1 1-e 1-e 0+e],[0 0 1 1-e 0+e 0+e],c2);patch([0 0 1 1-e 0+e 0+e],[0 1 1 1-e 1-e 0+e],c3);plot([0 1 1 0 0],[0 0 1 1 0]);
  wires:
  "p{3}"/1 -> mux/1
  mux/1 -> "pd{3,2}"/1

== system ball_and_plate_za_nn_2/NOE/Layer 3/LW{3,2} ==
  "ad{3,2}" : Inport  PortDimensions=10  SampleTime=0.001
      mask Display: e = 0.06;c1 = [120 230 180]/255;c2 = ([120 230 180]+0)/(256+128);c3 = ([120 230 180]+128)/(256+128);patch([0 1 1 0],[0 0 1 1],c1);patch([0 1 1 1-e 1-e 0+e],[0 0 1 1-e 0+e 0+e],c2);patch([0 0 1 1-e 0+e 0+e],[0 1 1 1-e 1-e 0+e],c3);plot([0 1 1 0 0],[0 0 1 1 0]);
  "IW{3,2}(1,:)'" : Constant  Value=[0.040413860274551162421463601504001417197287082672119140625;-0.922390700485416825671336482628248631954193115234375;-0.2847704915836410943796863648458383977413177490234375;-0.119375039110782898976736987606273032724857330322265625;-0.341439083972712775771896076548728160560131072998046875;-0.50733485064919781049042057929909788072109222412109375;0.8200616320720737206784178852103650569915771484375;-0.503983609435054713543422622024081647396087646484375;-0.57818123350426275930402653102646581828594207763671875;-0.64161556160537447368596986052580177783966064453125]
      mask Display: e = 0.06;c1 = [120 150 230]/255;c2 = ([120 150 230]+0)/383;c3 = ([120 150 230]+128)/383;patch([0 1 1 0],[0 0 1 1],c1);patch([0 1 1 1-e 1-e 0+e],[0 0 1 1-e 0+e 0+e],c2);patch([0 0 1 1-e 0+e 0+e],[0 1 1 1-e 1-e 0+e],c3);plot([0 1 1 0 0],[0 0 1 1 0]);disp('weights');
  "IW{3,2}(10,:)'" : Constant  Value=[0.346366935233423045570333442810806445777416229248046875;0.57982113783220901037651628939784131944179534912109375;0.57340249697952316854099308329750783741474151611328125;-0.63663622611961334651908828163868747651576995849609375;0.493057047298153694470101982005871832370758056640625;-0.61295474090280033241384671782725490629673004150390625;-0.307687812221070278173584711112198419868946075439453125;0.889968060640594416099702357314527034759521484375;0.218127843394698761603223147176322527229785919189453125;0.594582300739323610372366601950488984584808349609375]
      mask Display: e = 0.06;c1 = [120 150 230]/255;c2 = ([120 150 230]+0)/383;c3 = ([120 150 230]+128)/383;patch([0 1 1 0],[0 0 1 1],c1);patch([0 1 1 1-e 1-e 0+e],[0 0 1 1-e 0+e 0+e],c2);patch([0 0 1 1-e 0+e 0+e],[0 1 1 1-e 1-e 0+e],c3);plot([0 1 1 0 0],[0 0 1 1 0]);disp('weights');
  "IW{3,2}(2,:)'" : Constant  Value=[-0.247919268078307719616049098476651124656200408935546875;0.94436124925423892140230464065098203718662261962890625;0.9270543276709377611410900499322451651096343994140625;-0.392239860060123957108402237281552515923976898193359375;-0.28425051274919932442486469881259836256504058837890625;0.482043595032938976263636732255690731108188629150390625;0.055639342668838687178123336707358248531818389892578125;-0.596649201567405196300342140602879226207733154296875;0.30360672151137746421767360516241751611232757568359375;0.55585618915527390537789642621646635234355926513671875]
      mask Display: e = 0.06;c1 = [120 150 230]/255;c2 = ([120 150 230]+0)/383;c3 = ([120 150 230]+128)/383;patch([0 1 1 0],[0 0 1 1],c1);patch([0 1 1 1-e 1-e 0+e],[0 0 1 1-e 0+e 0+e],c2);patch([0 0 1 1-e 0+e 0+e],[0 1 1 1-e 1-e 0+e],c3);plot([0 1 1 0 0],[0 0 1 1 0]);disp('weights');
  "IW{3,2}(3,:)'" : Constant  Value=[0.7988372884423233788453444503829814493656158447265625;0.10264407291714987280339954622832010500133037567138671875;-0.30225989466886293843828070748713798820972442626953125;1.28639752379728378173240344040095806121826171875;0.555473538436132230344810523092746734619140625;0.258883734010433685934771119718789122998714447021484375;-0.6018171316378688739945346242166124284267425537109375;0.155025731162292956799575449622352607548236846923828125;0.1034283261229422823390677876886911690235137939453125;0.0768932827783828931611509460708475671708583831787109375]
      mask Display: e = 0.06;c1 = [120 150 230]/255;c2 = ([120 150 230]+0)/383;c3 = ([120 150 230]+128)/383;patch([0 1 1 0],[0 0 1 1],c1);patch([0 1 1 1-e 1-e 0+e],[0 0 1 1-e 0+e 0+e],c2);patch([0 0 1 1-e 0+e 0+e],[0 1 1 1-e 1-e 0+e],c3);plot([0 1 1 0 0],[0 0 1 1 0]);disp('weights');
  "IW{3,2}(4,:)'" : Constant  Value=[0.1877421742496100109942602784940390847623348236083984375;0.073772548326666242957116992329247295856475830078125;0.98389896042601099335200842688209377229213714599609375;0.1587567177918024763361160012209438718855381011962890625;-0.68414865746699071724634677593712694942951202392578125;0.90332478490211898236594834088464267551898956298828125;0.0626931921731869457037333859261707402765750885009765625;-0.047387286905901500333460063529855688102543354034423828125;-0.7018867120396026226814001347520388662815093994140625;-0.409896420558823637581014054376282729208469390869140625]
      mask Display: e = 0.06;c1 = [120 150 230]/255;c2 = ([120 150 230]+0)/383;c3 = ([120 150 230]+128)/383;patch([0 1 1 0],[0 0 1 1],c1);patch([0 1 1 1-e 1-e 0+e],[0 0 1 1-e 0+e 0+e],c2);patch([0 0 1 1-e 0+e 0+e],[0 1 1 1-e 1-e 0+e],c3);plot([0 1 1 0 0],[0 0 1 1 0]);disp('weights');
  "IW{3,2}(5,:)'" : Constant  Value=[0.34567979903814627373748180616530589759349822998046875;0.1689745227071446087574457806113059632480144500732421875;-0.65511477638029180781131799449212849140167236328125;-0.06799106151517965435093771020547137595713138580322265625;0.94811307052564597341870467062108218669891357421875;0.17434245159570094241274773594341240823268890380859375;0.399634533379687739707009086487232707440853118896484375;0.230065935698102574935575148629141040146350860595703125;-0.93213216556273181812031225490500219166278839111328125;0.8302746033940511249937799220788292586803436279296875]
      mask Display: e = 0.06;c1 = [120 150 230]/255;c2 = ([120 150 230]+0)/383;c3 = ([120 150 230]+128)/383;patch([0 1 1 0],[0 0 1 1],c1);patch([0 1 1 1-e 1-e 0+e],[0 0 1 1-e 0+e 0+e],c2);patch([0 0 1 1-e 0+e 0+e],[0 1 1 1-e 1-e 0+e],c3);plot([0 1 1 0 0],[0 0 1 1 0]);disp('weights');
  "IW{3,2}(6,:)'" : Constant  Value=[0.64148017317841821149926317957579158246517181396484375;0.371266902779530116873729639337398111820220947265625;-0.54654195876076572258028818396269343793392181396484375;-0.6314329269674636702092129780794493854045867919921875;-0.69913434240755389925681129170698113739490509033203125;0.70557959923069846208676381138502620160579681396484375;0.007333167928958259952632037226294414722360670566558837890625;-0.5018673974887419841905966677586548030376434326171875;0.5595800924386253871745111609925515949726104736328125;0.463373418118516344765822623230633325874805450439453125]
      mask Display: e = 0.06;c1 = [120 150 230]/255;c2 = ([120 150 230]+0)/383;c3 = ([120 150 230]+128)/383;patch([0 1 1 0],[0 0 1 1],c1);patch([0 1 1 1-e 1-e 0+e],[0 0 1 1-e 0+e 0+e],c2);patch([0 0 1 1-e 0+e 0+e],[0 1 1 1-e 1-e 0+e],c3);plot([0 1 1 0 0],[0 0 1 1 0]);disp('weights');
  "IW{3,2}(7,:)'" : Constant  Value=[-0.3769751902976870017170085702673532068729400634765625;0.74558407385953240353870796752744354307651519775390625;0.82763245776990423951957609460805542767047882080078125;-0.351946351905890908451368659370928071439266204833984375;-0.054512753614597987683598745434210286475718021392822265625;0.1042060761942014968095548965720809064805507659912109375;-0.3220293929206798910769293797784484922885894775390625;0.74298526277768084380426216739579103887081146240234375;0.478710071650852331259784477879293262958526611328125;0.65508440118354316350490762488334439694881439208984375]
      mask Display: e = 0.06;c1 = [120 150 230]/255;c2 = ([120 150 230]+0)/383;c3 = ([120 150 230]+128)/383;patch([0 1 1 0],[0 0 1 1],c1);patch([0 1 1 1-e 1-e 0+e],[0 0 1 1-e 0+e 0+e],c2);patch([0 0 1 1-e 0+e 0+e],[0 1 1 1-e 1-e 0+e],c3);plot([0 1 1 0 0],[0 0 1 1 0]);disp('weights');
  "IW{3,2}(8,:)'" : Constant  Value=[-0.724881375936054173081402041134424507617950439453125;-0.224228758994157562067783828751998953521251678466796875;-0.878991633763001711798779069795273244380950927734375;-0.34410970441512434003783482694416306912899017333984375;-0.796031048304059130060750248958356678485870361328125;-0.28685401288189849022813859846792183816432952880859375;0.597673707986199342911959320190362632274627685546875;0.204473374062566104480964668255182914435863494873046875;-0.12496619004476315628604510266086435876786708831787109375;-0.72977447209500478919608212891034781932830810546875]
      mask Display: e = 0.06;c1 = [120 150 230]/255;c2 = ([120 150 230]+0)/383;c3 = ([120 150 230]+128)/383;patch([0 1 1 0],[0 0 1 1],c1);patch([0 1 1 1-e 1-e 0+e],[0 0 1 1-e 0+e 0+e],c2);patch([0 0 1 1-e 0+e 0+e],[0 1 1 1-e 1-e 0+e],c3);plot([0 1 1 0 0],[0 0 1 1 0]);disp('weights');
  "IW{3,2}(9,:)'" : Constant  Value=[0.7355596049033739092237738077528774738311767578125;-0.61561420101332864351917351086740382015705108642578125;0.63945812650363631490790794487111270427703857421875;0.39810918430234931708611156864208169281482696533203125;0.45761704785750267898691845402936451137065887451171875;-0.01410886982849469777068218689919376629404723644256591796875;0.464929409371541313422682151212939061224460601806640625;-0.065512359979736423110097121025319211184978485107421875;-0.63074968859026470102691064312239177525043487548828125;-0.5151336803297141830881855639745481312274932861328125]
      mask Display: e = 0.06;c1 = [120 150 230]/255;c2 = ([120 150 230]+0)/383;c3 = ([120 150 230]+128)/383;patch([0 1 1 0],[0 0 1 1],c1);patch([0 1 1 1-e 1-e 0+e],[0 0 1 1-e 0+e 0+e],c2);patch([0 0 1 1-e 0+e 0+e],[0 1 1 1-e 1-e 0+e],c3);plot([0 1 1 0 0],[0 0 1 1 0]);disp('weights');
  Mux : Mux  Inputs=10
      mask Display: e = 0.06;c1 = [120 150 230]/255;c2 = ([120 150 230]+0)/383;c3 = ([120 150 230]+128)/383;patch([0 1 1 0],[0 0 1 1],c1);patch([0 1 1 1-e 1-e 0+e],[0 0 1 1-e 0+e 0+e],c2);patch([0 0 1 1-e 0+e 0+e],[0 1 1 1-e 1-e 0+e],c3);plot([0 1 1 0 0],[0 0 1 1 0]);disp('Mux');
  dotprod{1..10} (10 alike) : neural/Weight Functions/dotprod
  "lz{3,2}" : Outport
      mask Display: e = 0.06;c1 = [120 230 180]/255;c2 = ([120 230 180]+0)/(256+128);c3 = ([120 230 180]+128)/(256+128);patch([0 1 1 0],[0 0 1 1],c1);patch([0 1 1 1-e 1-e 0+e],[0 0 1 1-e 0+e 0+e],c2);patch([0 0 1 1-e 0+e 0+e],[0 1 1 1-e 1-e 0+e],c3);plot([0 1 1 0 0],[0 0 1 1 0]);
  wires:
  "IW{3,2}(1,:)'"/1 -> dotprod1/1
  "ad{3,2}"/1 -> dotprod1/2, dotprod2/2, dotprod3/2, dotprod4/2, dotprod5/2, dotprod6/2, dotprod7/2, dotprod8/2, dotprod9/2, dotprod10/2
  dotprod1/1 -> Mux/1
  "IW{3,2}(2,:)'"/1 -> dotprod2/1
  dotprod2/1 -> Mux/2
  "IW{3,2}(3,:)'"/1 -> dotprod3/1
  dotprod3/1 -> Mux/3
  "IW{3,2}(4,:)'"/1 -> dotprod4/1
  dotprod4/1 -> Mux/4
  "IW{3,2}(5,:)'"/1 -> dotprod5/1
  dotprod5/1 -> Mux/5
  "IW{3,2}(6,:)'"/1 -> dotprod6/1
  dotprod6/1 -> Mux/6
  "IW{3,2}(7,:)'"/1 -> dotprod7/1
  dotprod7/1 -> Mux/7
  "IW{3,2}(8,:)'"/1 -> dotprod8/1
  dotprod8/1 -> Mux/8
  "IW{3,2}(9,:)'"/1 -> dotprod9/1
  dotprod9/1 -> Mux/9
  "IW{3,2}(10,:)'"/1 -> dotprod10/1
  dotprod10/1 -> Mux/10
  Mux/1 -> "lz{3,2}"/1

== system ball_and_plate_za_nn_2/NOE/Layer 4/Delays 1 ==
  "p{4}" : Inport  PortDimensions=10  SampleTime=0.001
      mask Display: e = 0.06;c1 = [120 230 180]/255;c2 = ([120 230 180]+0)/(256+128);c3 = ([120 230 180]+128)/(256+128);patch([0 1 1 0],[0 0 1 1],c1);patch([0 1 1 1-e 1-e 0+e],[0 0 1 1-e 0+e 0+e],c2);patch([0 0 1 1-e 0+e 0+e],[0 1 1 1-e 1-e 0+e],c3);plot([0 1 1 0 0],[0 0 1 1 0]);
  mux : Mux  Inputs=1
      mask Display: e = 0.06;c1 = [120 150 230]/255;c2 = ([120 150 230]+0)/383;c3 = ([120 150 230]+128)/383;patch([0 1 1 0],[0 0 1 1],c1);patch([0 1 1 1-e 1-e 0+e],[0 0 1 1-e 0+e 0+e],c2);patch([0 0 1 1-e 0+e 0+e],[0 1 1 1-e 1-e 0+e],c3);plot([0 1 1 0 0],[0 0 1 1 0]);disp('Mux')
  "pd{4,3}" : Outport
      mask Display: e = 0.06;c1 = [120 230 180]/255;c2 = ([120 230 180]+0)/(256+128);c3 = ([120 230 180]+128)/(256+128);patch([0 1 1 0],[0 0 1 1],c1);patch([0 1 1 1-e 1-e 0+e],[0 0 1 1-e 0+e 0+e],c2);patch([0 0 1 1-e 0+e 0+e],[0 1 1 1-e 1-e 0+e],c3);plot([0 1 1 0 0],[0 0 1 1 0]);
  wires:
  "p{4}"/1 -> mux/1
  mux/1 -> "pd{4,3}"/1
